simulink model "RLC"  (R2020b)
settings: Solver=VariableStepAuto  StartTime=0.0  StopTime=simTime  RelTol=1e-3
undefined symbols (not defined in the file or in its folder): C, R, stepTime, V0, VF
settings Model: Creator=jvansick  LastModifiedBy=jvansick
settings SimscapeCC: SimscapeLogType=all

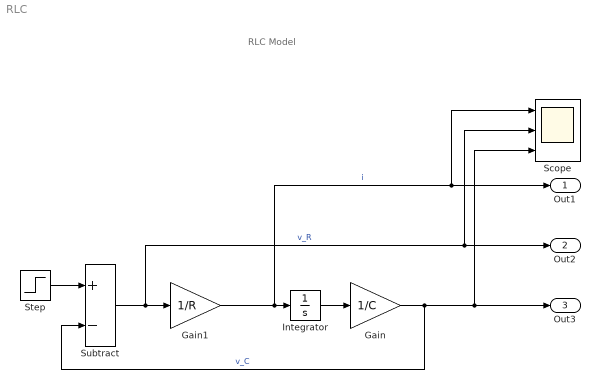
== system RLC ==
  note: RLC Model
  Gain : Gain  Gain=1/C
  Gain1 : Gain  Gain=1/R
  Integrator : Integrator
  Scope : Scope  NumInputPorts=3
  Step : Step  Time=stepTime  Before=V0  After=VF  SampleTime=0
  Subtract : Sum  Inputs=+-
  Out1 : Outport
  Out2 : Outport  Port=2
  Out3 : Outport  Port=3
  wires:
  Step/1 -> Subtract/1
  Integrator/1 -> Gain/1
  Gain/1 -> Scope/3, Out3/1, Subtract/2  "v_C"
  Subtract/1 -> Scope/2, Out2/1, Gain1/1  "v_R"
  Gain1/1 -> Scope/1, Out1/1, Integrator/1  "i"
